simulink model "first_cl"  (R2021a)
settings: Solver=VariableStepAuto  StartTime=0.0  StopTime=15  RelTol=1e-3
values from neighbouring files (symbols this model uses):
  disturbance = [0.05,0,0,0]    [ex2main.m]
  K = lqr_controller(sys)    [ex2main.m]
  sys = get_fullstate_system(params)    [ex2main.m]
  x_d = desired_state(theta_d, params)    [ex2main.m]
settings Model: Creator=martijndebeuf  LastModifiedBy=martijndebeuf
settings SolverCC: AlgebraicLoopSolver=TrustRegion
settings DebuggingCC: SFMachineParentedDataDiag=warning

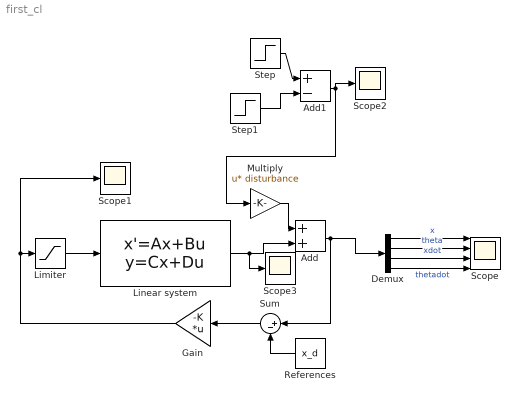
== system first_cl ==
  Add : Sum
  Add1 : Sum  Inputs=+-
  Demux : Demux
  Gain : Gain  Gain=-K  Multiplication=Matrix(K*u) (u vector)
  Limiter : Saturate  UpperLimit=3.5  LowerLimit=-3.5
  Linear system : StateSpace  A=sys.A  B=sys.B  C=eye(4)  D=zeros(4,1)  InitialCondition=initial_conditions'
  Multiply : Gain  Gain=disturbance  Multiplication=Matrix(u*K)
  References : Constant  Value=x_d
  Scope : Scope  NumInputPorts=4
  Scope1 : Scope
  Scope2 : Scope
  Scope3 : Scope
  Step : Step  Time=8  SampleTime=0
  Step1 : Step  Time=8.2  SampleTime=0
  Sum : Sum  Inputs=|+-
  wires:
  Sum/1 -> Gain/1
  References/1 -> Sum/2
  Demux/1 -> Scope/1  "x"
  Demux/2 -> Scope/2  "theta"
  Demux/3 -> Scope/3  "xdot"
  Demux/4 -> Scope/4  "thetadot"
  Limiter/1 -> Linear system/1
  Gain/1 -> Scope1/1, Limiter/1
  Step1/1 -> Add1/2
  Multiply/1 -> Add/1
  Add1/1 -> Scope2/1, Multiply/1
  Step/1 -> Add1/1
  Add/1 -> Sum/1, Demux/1
  Linear system/1 -> Scope3/1, Add/2
